simulink model "FOC_Controller"  (R2021a)
settings: Solver=FixedStepDiscrete  StartTime=0.0  StopTime=inf  FixedStep=4e-6  RelTol=1e-3
values from neighbouring files (symbols this model uses):
  FOC_bManualVdVq_C = Simulink.Parameter    [modeldata.m]
  FOC_iIdSP_C = Simulink.Parameter    [modeldata.m]
  FOC_kiPID_C = Simulink.Parameter    [modeldata.m]
  FOC_kpPID_C = Simulink.Parameter    [modeldata.m]
  FOC_uBusVoltage_C = Simulink.Parameter    [modeldata.m]
  FOC_uFindPosVd_C = Simulink.Parameter    [modeldata.m]
  FOC_uManualVd_C = Simulink.Parameter    [modeldata.m]
  FOC_uManualVq_C = Simulink.Parameter    [modeldata.m]
  Motor_bFindPosEnable_C = Simulink.Parameter    [modeldata.m]
  Motor_facTrq2Current_C = Simulink.Parameter    [modeldata.m]
  Motor_swtMode_C = Simulink.Parameter    [modeldata.m]
  Motor_tiFindPos_C = Simulink.Parameter    [modeldata.m]
  Motor_trqTorqueSetPoint_C = Simulink.Parameter    [modeldata.m]
  Position_degSetPoint_C = Simulink.Parameter    [modeldata.m]
  Position_kiPID_C = Simulink.Parameter    [modeldata.m]
  Position_kpPID_C = Simulink.Parameter    [modeldata.m]
  Position_nPIDMax_C = Simulink.Parameter    [modeldata.m]
  Speed_iPIDMax_C = Simulink.Parameter    [modeldata.m]
  Speed_kiPID_C = Simulink.Parameter    [modeldata.m]
  Speed_kpPID_C = Simulink.Parameter    [modeldata.m]
  Speed_nSetPoint_C = Simulink.Parameter    [modeldata.m]
  Speed_tiFilter_C = Simulink.Parameter    [modeldata.m]
libraries: simulink x11
(part 2 of 2)

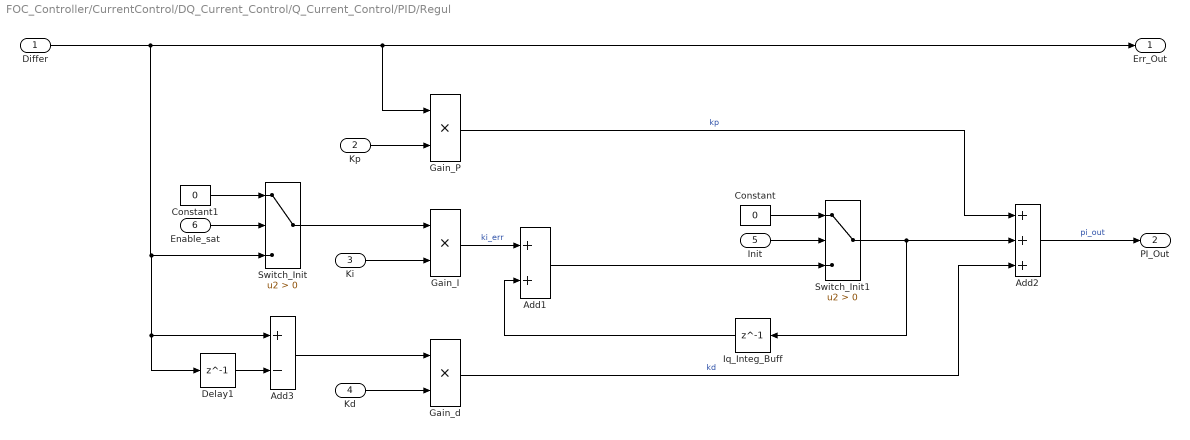
== system FOC_Controller/CurrentControl/DQ_Current_Control/Q_Current_Control/PID/Regul ==
  Differ : Inport
  Kp : Inport  Port=2
  Ki : Inport  Port=3
  Kd : Inport  Port=4
  Init : Inport  Port=5
  Enable_sat : Inport  Port=6
  Add1 : Sum  InputSameDT=on  SaturateOnIntegerOverflow=on  OutDataTypeStr=Inherit: Same as first input
  Add2 : Sum  Inputs=+++  InputSameDT=on  OutDataTypeStr=Inherit: Inherit via back propagation  SaturateOnIntegerOverflow=on
  Add3 : Sum  Inputs=+-  InputSameDT=on  SaturateOnIntegerOverflow=on
  Constant : Constant  Value=0  OutDataTypeStr=Inherit: Inherit via back propagation  SampleTime=-1
  Constant1 : Constant  Value=0  OutDataTypeStr=Inherit: Inherit via back propagation  SampleTime=-1
  Delay1 : Delay  DelayLength=1  InitialCondition=0
  Gain_I : Product  RndMeth=Zero  SaturateOnIntegerOverflow=on  OutDataTypeStr=Inherit: Same as first input
  Gain_P : Product  RndMeth=Zero  SaturateOnIntegerOverflow=on  OutDataTypeStr=Inherit: Same as first input
  Gain_d : Product  RndMeth=Zero  SaturateOnIntegerOverflow=on  OutDataTypeStr=Inherit: Same as first input
  Iq_Integ_Buff : Delay  DelayLength=1  InitialCondition=0
  Switch_Init : Switch  Criteria=u2 > Threshold
  Switch_Init1 : Switch  Criteria=u2 > Threshold  OutDataTypeStr=Inherit: Inherit via back propagation  InputSameDT=on
  Err_Out : Outport  InitialOutput=0  VectorParamsAs1DForOutWhenUnconnected=off
  PI_Out : Outport  Port=2  InitialOutput=0  VectorParamsAs1DForOutWhenUnconnected=off
  wires:
  Kd/1 -> Gain_d/2
  Gain_d/1 -> Add2/3  "kd"
  Add3/1 -> Gain_d/1
  Delay1/1 -> Add3/2
  Constant/1 -> Switch_Init1/1
  Add1/1 -> Switch_Init1/3
  Enable_sat/1 -> Switch_Init/2
  Constant1/1 -> Switch_Init/1
  Init/1 -> Switch_Init1/2
  Gain_I/1 -> Add1/1  "ki_err"
  Gain_P/1 -> Add2/1  "kp"
  Differ/1 -> Err_Out/1, Gain_P/1, Switch_Init/3, Add3/1, Delay1/1
  Add2/1 -> PI_Out/1  "pi_out"
  Switch_Init1/1 -> Iq_Integ_Buff/1, Add2/2
  Iq_Integ_Buff/1 -> Add1/2
  Kp/1 -> Gain_P/2
  Ki/1 -> Gain_I/2
  Switch_Init/1 -> Gain_I/1

== system FOC_Controller/CurrentControl/DQ_Current_Control/Q_Current_Control/PID/Saturation ==
  note: %大于最大值时，偏差仍为正，
      | 或小于最小值时，偏差仍为负，
      | 此时积分饱和限值%
  note: range[-AbsVmax~AbsVmax]
  Max : Inport
  Min : Inport  Port=2
  Err_in : Inport  Port=3
  Input : Inport  Port=4
  CompZero1 : simulink/Logic and Bit Operations/Compare To Zero  relop=<  OutDataTypeStr=boolean
  CompZero2 : simulink/Logic and Bit Operations/Compare To Zero  relop=>  OutDataTypeStr=boolean
  LogicalOperator1 : Logic  OutDataTypeStr=boolean
  LogicalOperator2 : Logic  OutDataTypeStr=boolean
  LogicalOperator3 : Logic  Operator=OR  OutDataTypeStr=boolean
  Sat : Subsystem
  Output : Outport  InitialOutput=0  VectorParamsAs1DForOutWhenUnconnected=off
  Enable_Sat : Outport  Port=2  InitialOutput=0  VectorParamsAs1DForOutWhenUnconnected=off
  wires:
  Max/1 -> Sat/1(Val_Max)
  Input/1 -> Sat/3(Val)
  Min/1 -> Sat/2(Val_Min)
  Sat/1(Val_Out) -> Output/1
  Sat/2(SatMax) -> LogicalOperator1/1
  Sat/3(SatMin) -> LogicalOperator2/1
  Err_in/1 -> CompZero1/1, CompZero2/1
  CompZero2/1 -> LogicalOperator1/2
  CompZero1/1 -> LogicalOperator2/2
  LogicalOperator1/1 -> LogicalOperator3/1
  LogicalOperator2/1 -> LogicalOperator3/2
  LogicalOperator3/1 -> Enable_Sat/1

== system FOC_Controller/PositionControl/Position_Control/PID/Saturation/Sat ==
  Val_Max : Inport
  Val_Min : Inport  Port=2
  Val : Inport  Port=3
  LogicalOperator2 : Logic  Operator=NOT  OutDataTypeStr=boolean
  Relational Operator : RelationalOperator  OutDataTypeStr=boolean  RndMeth=Nearest  InputSameDT=on
  Relational Operator1 : RelationalOperator  Operator=<=  OutDataTypeStr=boolean  RndMeth=Nearest  InputSameDT=on
  Switch_Inf : Switch  Criteria=u2 > Threshold  InputSameDT=on
  Switch_Sup : Switch  Criteria=u2 > Threshold  InputSameDT=on
  Val_Out : Outport  VectorParamsAs1DForOutWhenUnconnected=off
  SatMax : Outport  Port=2  InitialOutput=0  VectorParamsAs1DForOutWhenUnconnected=off
  SatMin : Outport  Port=3  InitialOutput=0  VectorParamsAs1DForOutWhenUnconnected=off
  wires:
  Switch_Inf/1 -> Val_Out/1
  Switch_Sup/1 -> Relational Operator/1, Switch_Inf/1
  Val_Max/1 -> Switch_Sup/1, Relational Operator1/1
  Val/1 -> Switch_Sup/3, Relational Operator1/2
  Val_Min/1 -> Switch_Inf/3, Relational Operator/2
  Relational Operator/1 -> LogicalOperator2/1, Switch_Inf/2
  Relational Operator1/1 -> SatMax/1, Switch_Sup/2
  LogicalOperator2/1 -> SatMin/1

== system FOC_Controller/SpeedControl/Speed_Control/PID/Saturation/Sat ==
  Val_Max : Inport
  Val_Min : Inport  Port=2
  Val : Inport  Port=3
  LogicalOperator2 : Logic  Operator=NOT  OutDataTypeStr=boolean
  Relational Operator : RelationalOperator  OutDataTypeStr=boolean  RndMeth=Nearest  InputSameDT=on
  Relational Operator1 : RelationalOperator  Operator=<=  OutDataTypeStr=boolean  RndMeth=Nearest  InputSameDT=on
  Switch_Inf : Switch  Criteria=u2 > Threshold  InputSameDT=on
  Switch_Sup : Switch  Criteria=u2 > Threshold  InputSameDT=on
  Val_Out : Outport  VectorParamsAs1DForOutWhenUnconnected=off
  SatMax : Outport  Port=2  InitialOutput=0  VectorParamsAs1DForOutWhenUnconnected=off
  SatMin : Outport  Port=3  InitialOutput=0  VectorParamsAs1DForOutWhenUnconnected=off
  wires:
  Switch_Inf/1 -> Val_Out/1
  Switch_Sup/1 -> Relational Operator/1, Switch_Inf/1
  Val_Max/1 -> Switch_Sup/1, Relational Operator1/1
  Val/1 -> Switch_Sup/3, Relational Operator1/2
  Val_Min/1 -> Switch_Inf/3, Relational Operator/2
  Relational Operator/1 -> LogicalOperator2/1, Switch_Inf/2
  Relational Operator1/1 -> SatMax/1, Switch_Sup/2
  LogicalOperator2/1 -> SatMin/1

== system FOC_Controller/CurrentControl/DQ_Current_Control/D_Current_Control/PID/Saturation/Sat ==
  Val_Max : Inport
  Val_Min : Inport  Port=2
  Val : Inport  Port=3
  LogicalOperator2 : Logic  Operator=NOT  OutDataTypeStr=boolean
  Relational Operator : RelationalOperator  OutDataTypeStr=boolean  RndMeth=Nearest  InputSameDT=on
  Relational Operator1 : RelationalOperator  Operator=<=  OutDataTypeStr=boolean  RndMeth=Nearest  InputSameDT=on
  Switch_Inf : Switch  Criteria=u2 > Threshold  InputSameDT=on
  Switch_Sup : Switch  Criteria=u2 > Threshold  InputSameDT=on
  Val_Out : Outport  VectorParamsAs1DForOutWhenUnconnected=off
  SatMax : Outport  Port=2  InitialOutput=0  VectorParamsAs1DForOutWhenUnconnected=off
  SatMin : Outport  Port=3  InitialOutput=0  VectorParamsAs1DForOutWhenUnconnected=off
  wires:
  Switch_Inf/1 -> Val_Out/1
  Switch_Sup/1 -> Relational Operator/1, Switch_Inf/1
  Val_Max/1 -> Switch_Sup/1, Relational Operator1/1
  Val/1 -> Switch_Sup/3, Relational Operator1/2
  Val_Min/1 -> Switch_Inf/3, Relational Operator/2
  Relational Operator/1 -> LogicalOperator2/1, Switch_Inf/2
  Relational Operator1/1 -> SatMax/1, Switch_Sup/2
  LogicalOperator2/1 -> SatMin/1

== system FOC_Controller/CurrentControl/DQ_Current_Control/Q_Current_Control/PID/Saturation/Sat ==
  Val_Max : Inport
  Val_Min : Inport  Port=2
  Val : Inport  Port=3
  LogicalOperator2 : Logic  Operator=NOT  OutDataTypeStr=boolean
  Relational Operator : RelationalOperator  OutDataTypeStr=boolean  RndMeth=Nearest  InputSameDT=on
  Relational Operator1 : RelationalOperator  Operator=<=  OutDataTypeStr=boolean  RndMeth=Nearest  InputSameDT=on
  Switch_Inf : Switch  Criteria=u2 > Threshold  InputSameDT=on
  Switch_Sup : Switch  Criteria=u2 > Threshold  InputSameDT=on
  Val_Out : Outport  VectorParamsAs1DForOutWhenUnconnected=off
  SatMax : Outport  Port=2  InitialOutput=0  VectorParamsAs1DForOutWhenUnconnected=off
  SatMin : Outport  Port=3  InitialOutput=0  VectorParamsAs1DForOutWhenUnconnected=off
  wires:
  Switch_Inf/1 -> Val_Out/1
  Switch_Sup/1 -> Relational Operator/1, Switch_Inf/1
  Val_Max/1 -> Switch_Sup/1, Relational Operator1/1
  Val/1 -> Switch_Sup/3, Relational Operator1/2
  Val_Min/1 -> Switch_Inf/3, Relational Operator/2
  Relational Operator/1 -> LogicalOperator2/1, Switch_Inf/2
  Relational Operator1/1 -> SatMax/1, Switch_Sup/2
  LogicalOperator2/1 -> SatMin/1

== stateflow chart FOC_Controller/ModeRegul/Chart ==
  state Initialization
    entry:
    bControlEnable = false;
    flagFindingPos = false;
  state Alignment
    entry:
    bControlEnable = false;
    flagFindingPos = true;
    during:holdtime = holdtime + DT;
  state Ready
    entry:
    bControlEnable = true;
  (default) -> Initialization
  Initialization -> Ready [order 2] : [FindPosEnable == false]
  Initialization -> Alignment [order 1] : [FindPosEnable == true]
      | {holdtime=0;}
  Alignment -> Ready : [holdtime > Motor_tiFindPos_C]...
      | {flagFindingPos=false;
      | calibration_angle = measure_angle;}
  data: FindPosEnable input; holdtime local uint16; flagFindingPos output boolean; bControlEnable output boolean; Motor_tiFindPos_C input; measure_angle input; DT input; calibration_angle output uint16
